simulink model "garmi_whole_body_ufic"  (R2022b)
settings: Solver=ode1  StartTime=0.0  StopTime=40  FixedStep=.001  RelTol=1e-3  AbsTol=1e-3
libraries: slpidlib x1, simulink x1
(part 1 of 2)
settings Model: Creator=ge85xev  LastModifiedBy=ge85xev
settings SolverCC: AutoScaleAbsTol=off
settings ModelReferenceCC: EnableRefExpFcnMdlSchedulingChecks=on

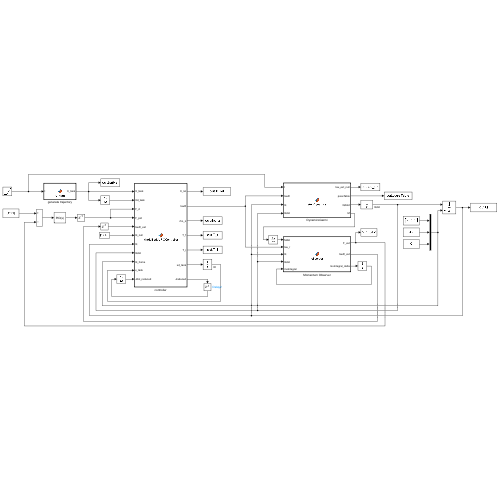
[thumbnail: Simulink's stored preview of the top-level diagram]
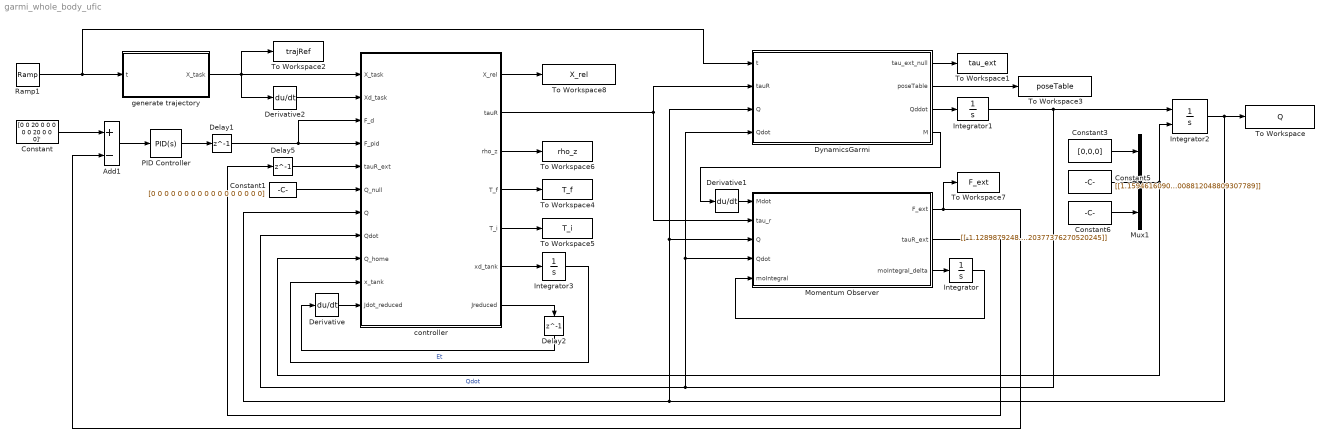
== system garmi_whole_body_ufic ==
  Add1 : Sum  Inputs=+-
  Constant : Constant  Value=[0 0 20 0 0 0 0 0 20 0 0 0]'
  Constant1 : Constant  Value=[0 0 0 0 0 0 0 0 0 0 0 0 0 0 0 0 0]
  Constant3 : Constant  Value=[0,0,0]
  Constant5 : Constant  Value=[[1.159461609037299, -1.6000122252681799, -0.05584684541350855, -2.1649581944754175, -2.649529466629028, 2.466730273079475, -0.008812048809307789]]
  Constant6 : Constant  Value=[[-1.1289879248603267, -1.526043571178735, 0.1314950197577818, -2.0453876018029984, 2.3706213790056045, 2.5849102800687156, 0.20377376270520245]]
  Delay1 : Delay  DelayLength=1  InitialCondition=zeros(12,1)
  Delay2 : Delay  DelayLength=1  InitialCondition=zeros(12,16)
  Delay5 : Delay  DelayLength=1  InitialCondition=zeros(16,1)
  Derivative : Derivative
  Derivative1 : Derivative
  Derivative2 : Derivative
  DynamicsGarmi : MATLAB Function  TreatAsAtomicUnit=on  SystemSampleTime=0.001
  Integrator : Integrator  InitialCondition=zeros(16,1)
  Integrator1 : Integrator  InitialCondition=[0,0,0,0,0,0,0,0,0,0,0,0,0,0,0,0,0]
  Integrator2 : Integrator  InitialConditionSource=external  InitialCondition=[0.942613,-1.37299,-0.0288793,-1.84589,0.131607,1.92806,-0.40]
  Integrator3 : Integrator  InitialCondition=[0.01;0.01]
  Momentum Observer : MATLAB Function  TreatAsAtomicUnit=on  SystemSampleTime=0.001
  Mux1 : Mux  Inputs=3
  PID Controller : slpidlib/PID Controller  Controller=PID  Form=Parallel  TimeDomain=Continuous-time  UseExternalTs=off  SampleTime=-1  IntegratorMethod=Forward Euler  FilterMethod=Forward Euler  ControllerParametersSource=internal  P=0.1  I=0.0  UseKiTs=off  D=0.0  N=100  UseFilter=on  TunerSelectOption=Transfer Function Based (PID Tuner App)  InitialConditionSource=internal  InitialConditionForIntegrator=0  InitialConditionForFilter=0  DifferentiatorICPrevScaledInput=0  ExternalReset=none  TrackingMode=off  Kt=1  LimitOutput=off  SatLimitsSource=internal  UpperSaturationLimit=inf  LowerSaturationLimit=-inf  LinearizeAsGain=on  AntiWindupMode=none  Kb=1  LimitIntegrator=off  UpperIntegratorSaturationLimit=inf  LowerIntegratorSaturationLimit=-inf  POutMin=[]  POutMax=[]  IOutMin=[]  IOutMax=[]  DOutMin=[]  DOutMax=[]  NOutMin=[]  NOutMax=[]  SumOutMin=[]  SumOutMax=[]  SaturationOutMin=[]  SaturationOutMax=[]  PParamMin=[]  PParamMax=[]  IParamMin=[]  IParamMax=[]  DParamMin=[]  DParamMax=[]  NParamMin=[]  NParamMax=[]  KbParamMin=[]  KbParamMax=[]  KtParamMin=[]  KtParamMax=[]  KbOutMin=[]  KbOutMax=[]  KtOutMin=[]  KtOutMax=[]  IntegratorOutMin=[]  IntegratorOutMax=[]  FilterOutMin=[]  FilterOutMax=[]  SumI1OutMin=[]  SumI1OutMax=[]  SumI2OutMin=[]  SumI2OutMax=[]  SumI3OutMin=[]  SumI3OutMax=[]  SumI4OutMin=[]  SumI4OutMax=[]  SumDOutMin=[]  SumDOutMax=[]  DifferentiatorOutMin=[]  DifferentiatorOutMax=[]  FilterDiffOutCoefMin=[]  FilterDiffOutCoefMax=[]  ReciprocalOutMin=[]  ReciprocalOutMax=[]  SumDenOutMin=[]  SumDenOutMax=[]  SumNumOutMin=[]  SumNumOutMax=[]  DivideOutMin=[]  DivideOutMax=[]  UdiffTsProdOutMin=[]  UdiffTsProdOutMax=[]  NTsProdOutMin=[]  NTsProdOutMax=[]  UintegralTsProdOutMin=[]  UintegralTsProdOutMax=[]  UngainTsProdOutMin=[]  UngainTsProdOutMax=[]  ClampingZeroOutDataTypeStr=Inherit: Inherit via back propagation  ClampingZeroOutMin=[]  ClampingZeroOutMax=[]  FilterDenConstantOutDataTypeStr=Inherit: Inherit via back propagation  FilterDenConstantOutMin=[]  FilterDenConstantOutMax=[]  PCopyOutDataTypeStr=Inherit: Inherit via back propagation  PCopyOutMin=[]  PCopyOutMax=[]  NCopyOutDataTypeStr=Inherit: Inherit via back propagation  NCopyOutMin=[]  NCopyOutMax=[]  IntegratorContinuousStateAttributes=''  IntegratorStateMustResolveToSignalObject=off  IntegratorRTWStateStorageClass=Auto  FilterContinuousStateAttributes=''  FilterStateMustResolveToSignalObject=off  FilterRTWStateStorageClass=Auto  ParallelPVariant=InternalParameters  IdealPVariant=Disabled  IVariant=InternalParameters  DVariant=InternalParameters  IntegratorVariant=Continuous  SatVariant=Disabled  AWVariant=Passthrough  PCopyVariant=Disabled  TRVariant=Disabled  FdbkBlocksVariant=Forward  IdealPFdbkVariant=Disabled  SatFdbkVariant=Disabled  DerivativeFilterVariant=ContFilter  NVariant=InternalParameters  NCopyVariant=Disabled  FilterICVariant=InternalICsFilter  IntegratorICVariant=InternalICs  ExternalResetVariant=Disabled  TRSumVariant=Passthrough  SumFdbkVariant=Disabled  SumVariant=Sum_PID  TsampFilterVariant=InternalTs  TsampNgainVariant=Passthrough  TsampIntegralVariant=Passthrough  ExternalSaturationOutDataTypeStr=Inherit: Same as second input
  Ramp1 : simulink/Sources/Ramp  slope=1  start=0  InitialOutput=0
  To Workspace : ToWorkspace  VariableName=Q  SaveFormat=Timeseries  SampleTime=-1
  To Workspace1 : ToWorkspace  VariableName=tau_ext  SaveFormat=Timeseries  SampleTime=-1
  To Workspace2 : ToWorkspace  VariableName=trajRef  SaveFormat=Timeseries  SampleTime=-1
  To Workspace3 : ToWorkspace  VariableName=poseTable  SaveFormat=Timeseries  SampleTime=-1
  To Workspace4 : ToWorkspace  VariableName=T_f  SaveFormat=Timeseries  SampleTime=-1
  To Workspace5 : ToWorkspace  VariableName=T_i  SaveFormat=Timeseries  SampleTime=-1
  To Workspace6 : ToWorkspace  VariableName=rho_z  SaveFormat=Timeseries  SampleTime=-1
  To Workspace7 : ToWorkspace  VariableName=F_ext  SaveFormat=Timeseries  SampleTime=-1
  To Workspace8 : ToWorkspace  VariableName=X_rel  SaveFormat=Timeseries  SampleTime=-1
  controller : MATLAB Function  TreatAsAtomicUnit=on
  generate trajectory : MATLAB Function  TreatAsAtomicUnit=on
  wires:
  Integrator1/1 -> Integrator2/1, DynamicsGarmi/4(Qdot), Momentum Observer/4(Qdot), controller/8(Qdot)  "Qdot"
  Integrator2/1 -> To Workspace/1, controller/7(Q), DynamicsGarmi/3(Q), Momentum Observer/3(Q)
  Mux1/1 -> Integrator2/2, controller/9(Q_home)
  Constant3/1 -> Mux1/1
  Constant5/1 -> Mux1/2
  Constant6/1 -> Mux1/3
  Derivative/1 -> controller/11(Jdot_reduced)
  controller/7(Jreduced) -> Delay2/1
  DynamicsGarmi/3(Qddot) -> Integrator1/1
  generate trajectory/1(X_task) -> To Workspace2/1, controller/1(X_task), Derivative2/1
  Momentum Observer/3(moIntegral_delta) -> Integrator/1
  Integrator/1 -> Momentum Observer/5(moIntegral)
  DynamicsGarmi/4(M) -> Derivative1/1
  Derivative1/1 -> Momentum Observer/1(Mdot)
  Delay2/1 -> Derivative/1
  Constant/1 -> Add1/1
  Add1/1 -> PID Controller/1
  Momentum Observer/2(tauR_ext) -> Delay5/1
  Delay5/1 -> controller/5(tauR_ext)
  controller/2(tauR) -> DynamicsGarmi/2(tauR), Momentum Observer/2(tau_r)
  Momentum Observer/1(F_ext) -> To Workspace7/1, Add1/2
  DynamicsGarmi/1(tau_ext_null) -> To Workspace1/1
  Delay1/1 -> controller/3(F_d), controller/4(F_pid)
  PID Controller/1 -> Delay1/1
  controller/6(xd_tank) -> Integrator3/1
  Integrator3/1 -> controller/10(x_tank)  "Et"
  Derivative2/1 -> controller/2(Xd_task)
  controller/4(T_f) -> To Workspace4/1
  controller/5(T_i) -> To Workspace5/1
  DynamicsGarmi/2(poseTable) -> To Workspace3/1
  Constant1/1 -> controller/6(Q_null)
  Ramp1/1 -> DynamicsGarmi/1(t), generate trajectory/1(t)
  controller/3(rho_z) -> To Workspace6/1
  controller/1(X_rel) -> To Workspace8/1

== matlab function garmi_whole_body_ufic/generate trajectory ==
  data: t input; X_task output
function X_task = refPath(t)
    % Generates a circular trajectory for the right arm in the XY plane
    % using screw representation, while keeping the left arm's pose unchanged.
    %
    % Input:
    %   t      - Current time
    %
    % Output:
    %   X_task - 6x2 matrix representing [Right Arm Screw Pose, Left Arm Screw Pose]

    % Define parameters
    radius = 0.1;                  % Circle radius
    center = [0.0,0.0,0.0];        % Circle center (x, y, z)
    frequency = 0.1;               % Frequency in Hz
    go_down = 0.15;

    % Compute circular trajectory for right arm in XY plane
    theta = 2 * pi * frequency * t;
    x_r = center(1) + radius * (1-cos(theta));
    y_r = center(2) - radius * sin(theta);
    z_r = center(3) - go_down*(1 - exp(-0.5 * t));

    x_l = center(1) + radius * (1-cos(theta));
    y_l = center(2) + radius * sin(theta);
    z_l = center(3) - go_down*(1 - exp(-0.5 * t));

    % Construct the output 6x2 matrix
    X_task = [x_r, y_r, z_r, 0, 0, 0, x_l, y_l, z_l, 0, 0, 0]';
end

== matlab function garmi_whole_body_ufic/DynamicsGarmi ==
  data: tau_ext_null output; poseTable output; t input; tauR input; Q input; Qdot input; Qddot output; M output
function  [tau_ext_null, poseTable, Qddot,M] = stepDynamics(t, tauR, Q, Qdot)
X = [pose_arm(Q, 8, true), pose_arm(Q, 8, false)];
% Compute Whole Body Jacobian for right and left arm
Jwb_right = JacobianWholeBody(Q,8,true);
Jwb_left = JacobianWholeBody(Q,8,false);
Jwb = [Jwb_right;Jwb_left];
Xdot = Jwb*Qdot;

% Compute whole body dynamics  model for the model based control.
[M, C, G] = computeDynamics(Q, Qdot);

[f_ext_task, tau_ext_null, poseTable] = dist(X, Xdot, t);

% watch this video to learn how to drive these equations:
%  https://www.youtube.com/watch?v=C1cb03fYkxk

% Nonholomonic contriant matrix:
A = [-sin(Q(3)), cos(Q(3)), 0, zeros(1,14)];
Adot = [-Qdot(3)*cos(Q(3)), -Qdot(3)*sin(Q(3)), 0, zeros(1,14)];

% Computations for reduced order dynamics with the nonholonimic constraint
D = [cos(Q(3)), sin(Q(3)), zeros(1,15);zeros(15,2),eye(15,15)]; % D is auxilary and arbitrary matrix to make a non-singular square constriant matrix
Ddot = [-Qdot(3)*sin(Q(3)), Qdot(3)*cos(Q(3)), zeros(1,15);zeros(15,2),zeros(15,15)];
A_D = [A;D]; % This square matrix will be used to reduce the dynamics due to its constriant.
inverse_A_D = [-sin(Q(3)), cos(Q(3)), zeros(1,15);cos(Q(3)), sin(Q(3)), zeros(1,15);zeros(15,2),eye(15,15)]; % since the D matrix is easy, we analatically inverse it
E = inverse_A_D(:,1); % if the number of the constraints are M, then the first M columns are E
F = inverse_A_D(:,2:end); % if the number of the constraints are M, then the rest of columns (N-M) are F
v = D * Qdot;  % pseudo velocities that are used as the reduced generalized coordinates of the system.

% map external force to reduced external torques:
tau_ext = (Jwb_right*F)'*f_ext_task(1:6) + (Jwb_left*F)'*f_ext_task(7:12) + tau_ext_null;

% Compute reduced dynamics
M_reduced = F'*M*F; % Reduced mass matrix of the system.
vdot = M_reduced \ (tauR + tau_ext - F'*C*F*v - F'*G + F'*M*(E*Adot + F*Ddot)*F*v);  % reduced dynamics of the system.
Qddot = F*vdot - (E*Adot + F*Ddot)*F*v;  % convert the reduced coordinates to the origin generalized coordinate.

    function crossMatrix = crossOperator(vec)
        crossMatrix = [0, -vec(3), vec(2); vec(3), 0, -vec(1); -vec(2), vec(1), 0];
    end

    function T = DHmatrix(q, i)
        % Define DH parameters for each link
        l = 0.1; % Tool length
        d = [0.333, 0, 0.316, 0, 0.384, 0, 0, 0.107+l];
        a = [0, 0, 0, 0.0825, -0.0825, 0, 0.088, 0];
        alpha = [0, -pi/2, pi/2, pi/2, -pi/2, pi/2, pi/2, 0];
        q_ext = [q; 0];

        % DH Transformation matrix for the current joint
        ct = cos(q_ext(i));
        st = sin(q_ext(i));
        ca = cos(alpha(i));
        sa = sin(alpha(i));

        T = [ ct, -st, 0, a(i);
            st * ca, ct * ca, -sa, -sa * d(i);
            st * sa, ct * sa, ca, ca * d(i);
            0, 0, 0, 1];  % calculate denavit hartenberg matrix
    end

    function T_total = FK(Q, index, isRightArm)
        % Extract pose components
        x = Q(1);
        y = Q(2);
        theta = Q(3);

        % Select the correct segment of Q based on isRightArm
        if isRightArm
            q_arm = Q(4:10); % Right arm joint angles
        else
            q_arm = Q(11:17); % Left arm joint angles
        end

        % --- Parameters Definition ---
        % Base dimensions
        width = 0.75; % X-direction (width)
        height = 0.2; % Y-direction (height)
        depth = 0.75; % Z-direction (depth)

        % Wheel parameters
        wheelRadius = height / 2; % Radius of the wheels

        % Spine length along the Z-axis and offset along the Y-axis
        spineHeight = 1.05;
        spineOffset = 0.1;

        % Shoulder width along the X-axis
        shoulderWidth = 0.4;

        % Rotation matrix to compensate the installation of Franka Arms on Garmi
        % torso
        if isRightArm
            beta = pi/2.0; % Rotation about Y axis
            gamma = pi/2.0; % Rotation about Z axis
            shoulderPose = [spineOffset , -shoulderWidth/2, height+ spineHeight]; % shoulderWidth/2 m to the right
        else
            beta = pi/2.0; % Rotation about Y axis
            gamma = -pi/2.0; % Rotation about Z axis
            shoulderPose = [spineOffset  , shoulderWidth/2, height+ spineHeight]; % shoulderWidth/2 m to the left
        end

        % Transformation matrix for the base of garmi
        T_mobile_base = [cos(theta), -sin(theta), 0 , x;
            sin(theta), cos(theta) , 0 , y;
            0,          0,           1 , 0;
            0,          0,           0 ,1];
        % Transformation matrix for the shoulder pose
        Tshoulder = [1, 0, 0, shoulderPose(1);
            0, 1, 0, shoulderPose(2);
            0, 0, 1, shoulderPose(3);
            0, 0, 0, 1];

        % Transformation matrix for the Garmi wall-mount arm installation
        Ty = [cos(beta), 0, sin(beta), 0;
            0, 1, 0, 0;
            -sin(beta), 0, cos(beta), 0;
            0, 0, 0, 1];
        Tz = [cos(gamma), -sin(gamma), 0, 0;
            sin(gamma), cos(gamma), 0, 0;
            0, 0, 1, 0;
            0, 0, 0, 1];

        % Transformation of the arm_base to the universal frame
        Ti = T_mobile_base* Tshoulder * Ty * Tz;

        for arm_id = 1:index
            Ti = Ti * DHmatrix(q_arm, arm_id); % apply rotation matrix to compensate for arm configuration
        end

        T_total = Ti;
    end

    function X = pose_arm(Q, index, isRightArm)
        % init pose vector:
        X = zeros(6,1);

        % Compute the transformation matrix for the specified configuration
        T_idx = FK(Q, index, isRightArm);

        % Extract the rotation matrix from the transformation matrix
        R = T_idx(1:3, 1:3);

        % Convert the rotation matrix to an axis-angle representation
        angle = acos((trace(R) - 1) / 2);
        if angle ~= 0
            % Ensure the angle is non-zero to avoid division by zero
            axis = [R(3,2) - R(2,3); R(1,3) - R(3,1); R(2,1) - R(1,2)] / (2*sin(angle));
            % Normalize the axis to ensure it's a unit vector
            axis = axis / norm(axis);
        else
            % Handle the case of a zero angle, implying no rotation or a full rotation
            axis = [0; 0; 1]; % Default axis if no rotation is present
        end

        % return pose vector
        X(1:3)= T_idx(1:3,4);
        X(4:6) = angle * axis;
    end

    function positions = getJointsPositions(Q, isRightArm)
        positions = zeros(3, 8); % Initialize positions matrix

        for arm_id = 1:8
            T = FK(Q, arm_id, isRightArm);
            positions(:, arm_id) = T(1:3, 4); % Extract and store the position
        end
    end

    function Jacobian = JacobArm(Q, index, isRightArm)

        % Initialize the Jacobian matrix with zeros
        Jacobian = zeros(6, 7);

        % Compute FK up to the specified joint index
        T_joint_index = FK(Q, index, isRightArm);
        P_joint_index = T_joint_index(1:3, 4); % Extract the position vector of the joint at the specified index

        for arm_id = 1:index-1  % count joint positions up to one before the target joint.
            % Compute the transformation matrix up to the current joint
            Ti = FK(Q, arm_id, isRightArm);

            % Extract the joint axis of the current joint
            P_i = Ti(1:3, 4);

            % Calculate the columns of the Jacobian matrix
            z_current = Ti(1:3, 3);
            p_diff = P_joint_index - P_i;

            % Update the Jacobian matrix
            % Linear velocity part
            Jacobian(1:3, arm_id) = cross(z_current, p_diff);
            % Angular velocity part
            Jacobian(4:6, arm_id) = z_current;
        end
    end

    function Jacobian = JacobBody(Q, index, isRightArm)

        % Compute FK up to the specified joint index
        T_joint_index = FK(Q, index, isRightArm);

        % Extract the position of the joint at the specified index
        % in absolute frame relative to robot base center.
        P_joint_index = T_joint_index(1:3, 4) - [Q(1),Q(2),0]';

        % Nonholonomic matrix setup (assuming linear and angular velocity command scenario)
        nonholonomicMatrix = [1, 0, 0 ; 0, 1, 0 ; 0, 0, 0 ; 0, 0, 0 ; 0, 0, 0 ; 0, 0, 1];
        %nonholonomicMatrix = [cos(pose(3)), 0; sin(pose(3)), 0; 0, 0; 0, 0; 0, 0; 0, 1];

        % Calculate the Jacobian for the platform
        crossProdMatrix = crossOperator(P_joint_index);
        JacobianPlatform = [eye(3), -crossProdMatrix; zeros(3, 3), eye(3)];

        % Apply the nonholonomic constraints to the platform Jacobian
        Jacobian = JacobianPlatform * nonholonomicMatrix;
    end

    function J_wb = JacobianWholeBody(Q, index, isRightArm)
        J_arm = JacobArm(Q, index, isRightArm);
        J_body = JacobBody(Q, index, isRightArm);
        if isRightArm
            % Assemble the whole-body Jacobian for the right side
            J_wb = [J_body, J_arm, zeros(6, 7)];
        else
            % Assemble the whole-body Jacobian for the left side
            J_wb = [J_body, zeros(6, 7), J_arm];
        end
    end

    function jacobian = JacobArm_cg(Q, index, isRightArm)
        jacobian = zeros(6, 7); % Pre-allocate for speed
        linkCoMs = zeros(3, 7);

        % Updated CoM for each link (expressed as offsets from the link frame)
        linkCoMs = [0, -0.0256, 0.00652, -0.0472, -0.00402, 0.1263, 0.1;
            -5.844e-9, -0.323, 0.0228, 0.000919, 0.0770, -0.0410, 0.00290;
            -0.391, 0.0706, -0.0701, 0.0287, -0.376, -0.0109, 0.0272];

        T_mi = FK(Q, index, isRightArm);
        R_mi = T_mi(1:3,1:3);
        joint_position_before_mi = T_mi(1:3,4);
        r_mi_abs = joint_position_before_mi + R_mi * linkCoMs(:, index); % center of mass position of link i in global frame relative to global frame

        for joint_number = 1:index
            Ti = FK(Q,joint_number,isRightArm);
            joint_position = Ti(1:3,4);
            joint_axis = Ti(1:3,3);  % frame z axis is equivalent to the joint axis vector.

            jacobian(1:3, joint_number) = cross(joint_axis, (r_mi_abs - joint_position));
            jacobian(4:6, joint_number) = joint_axis;
        end
    end

    function Jacobian = JacobBody_cg(Q, index, isRightArm)

        % Updated CoM for each link (expressed as offsets from the link frame)
        linkCoMs = [0, -0.0256, 0.00652, -0.0472, -0.00402, 0.1263, 0.1;
            -5.844e-9, -0.323, 0.0228, 0.000919, 0.0770, -0.0410, 0.00290;
            -0.391, 0.0706, -0.0701, 0.0287, -0.376, -0.0109, 0.0272];

        % Compute FK up to the specified joint index
        T_mi = FK(Q, index, isRightArm);
        R_mi = T_mi(1:3,1:3);
        joint_position_before_cg = T_mi(1:3,4);
        r_mi_abs = joint_position_before_cg + R_mi * linkCoMs(:, index); % center of mass position of link i in global frame


        r_mi_abs_rel = r_mi_abs - [Q(1),Q(2),0]'; % center of mass position of link i relative to mobile base frame

        % Nonholonomic matrix setup (assuming linear and angular velocity command scenario)
        nonholonomicMatrix = [1, 0, 0 ; 0, 1, 0 ; 0, 0, 0 ; 0, 0, 0 ; 0, 0, 0 ; 0, 0, 1];

        % Calculate the Jacobian for the platform
        crossProdMatrix = crossOperator(r_mi_abs_rel);
        JacobianPlatform = [eye(3), -crossProdMatrix; zeros(3, 3), eye(3)];

        % Apply the nonholonomic constraints to the platform Jacobian
        Jacobian = JacobianPlatform * nonholonomicMatrix;
    end

    function J_wb = JacobianWholeBody_cg(Q, index, isRightArm)
        J_arm = JacobArm_cg(Q, index, isRightArm);
        J_body = JacobBody_cg(Q, index, isRightArm);
        if isRightArm
            % Assemble the whole-body Jacobian for the right side
            J_wb = [J_body, J_arm, zeros(6, 7)];
        else
            % Assemble the whole-body Jacobian for the left side
            J_wb = [J_body, zeros(6, 7), J_arm];
        end
    end

% Dynamics
    function [M, C, G] = computeDynamics(Q, Qdot)
        % Dynamic parameters
        g = [0; 0; -9.81];
        payloadMass = 0.77;

        % Updated mass for each link
        linkMasses = [4.07, 5.996, 0.570, 3.083, 3.616, 1.435, 0.453 + payloadMass];

        % Updated inertia matrices for each link, approximated and written inline
        linkInertia = zeros(3, 21);
        linkInertia(:, 1:3) = [4.47e-6, 0, 0; 0, 4.47e-6, -5.61e-10; 0, -5.61e-10, 2.00e-6]; % Link 1
        linkInertia(:, 4:6) = [0.0465, -0.00338, 0.000748; -0.00338, 0.00243, 0.00980; 0.000748, 0.00980, 0.0445]; % Link 2
        linkInertia(:, 7:9) = [0.0504, 0.00248, -0.0118; 0.00248, 0.0525, 0.00747; -0.0118, 0.00747, 0.00817]; % Link 3
        linkInertia(:, 10:12) = [0.0308, 0.00732, 0.000194; 0.00732, 0.00278, 0.00101; 0.000194, 0.00101, 0.0329]; % Link 4
        linkInertia(:, 13:15) = [0.0511, -0.000984, -0.00223; -0.000984, 0.0472, 0.00346; -0.00223, 0.00346, 0.00475]; % Link 5
        linkInertia(:, 16:18) = [0.00823, 0.00463, -0.00127; 0.00463, 0.0187, 0.00110; -0.00127, 0.00110, 0.0144]; % Link 6
        linkInertia(:, 19:21) = [0.00378, -3.27e-5, -0.000200; -3.27e-5, 0.00368, -0.000602; -0.000200, -0.000602, 0.000122]; % Link 7


        % Mass and Inertia parameters for mobile base
        baseMass = 50;
        baseInertia = 15;

        M = zeros(17, 17);
        C = zeros(17, 17);
        G = zeros(17, 1);

        % Arm dynamics computation for both arms
        for arm = 1:2 % 1 for right arm, 2 for left arm
            for arm_id = 1:7
                Tcg = FK(Q, arm_id, arm == 1);
                Rcg = Tcg(1:3, 1:3);
                Jwb_cg = JacobianWholeBody_cg(Q, arm_id, arm == 1);
                linkmass = linkMasses(arm_id);
                InertiaMatrix = reshape(linkInertia(:, 3*arm_id-2:3*arm_id), 3, 3);

                mass_link = zeros(6, 6);
                mass_link(1:3, 1:3) = linkmass * eye(3);
                mass_link(4:6, 4:6) = Rcg * InertiaMatrix * Rcg';

                Jwb_cg_v = Jwb_cg(1:3, :);

                M = M + Jwb_cg' * mass_link * Jwb_cg;
                G = G - linkmass * Jwb_cg_v' * g;
            end
            C = zeros(17, 1);
        end

        JacobBase = [eye(3),zeros(3,7),zeros(3,7)];  % jacobian of mobile base vb = JacobBase*Qdot
        % Base dynamics
        M = M + JacobBase'*diag([baseMass, baseMass, baseInertia])*JacobBase;
        G = G + zeros(17,1);
        C = C + zeros(17, 17);
    end

    function [f_ext_task, tau_ext_null, poseTable] = dist(X, Xdot, t)
        % Computes external force and torque if the arms are in contact with the table.

        % Table parameters
        poseTable = [1.20;0.0;1.0 - (t > 20)];
        widthTable = 0.5;
        lengthTable = 0.8;

        % Contact model
        stiffness = 1e4;
        damping = 1000;

        % Initialize forces
        f_ext_task = zeros(12,1);

        % Check contact for both arms
        for i = 1:2
            in_x_range = abs(X(i*6-5) - poseTable(1)) <= widthTable / 2;
            in_y_range = abs(X(i*6-4) - poseTable(2)) <= lengthTable / 2;
            in_contact = (X(i*6-3) <= poseTable(3)) && in_x_range && in_y_range;

            if in_contact
                penetration = poseTable(3) - X(i*6-3);
                f_ext_task(i*6-3) = stiffness * penetration - damping * Xdot(i*6-3);
            end
        end

        % External torques
        gain_x = -0.0;  % -20
        gain_theta = 0.0;  % 20.0
        now_start = 1.0;
        tau_ext_null = zeros(16,1);

        tau_ext_null(1) = (t > now_start && t <= now_start + 2.5) * gain_x ...
            - (t > now_start + 2.5 && t <= now_start + 5.0) * gain_x;

        tau_ext_null(2) = (t > now_start + 10 && t <= now_start + 12.5) * gain_theta ...
            - (t > now_start + 12.5 && t <= now_start + 15.0) * gain_theta;
    end
end
